simulink model "FourFlexibleBarsFreeAug"  (R2025b)
settings: Solver=VariableStepAuto  StartTime=0.0  StopTime=10.0  RelTol=1e-3
undefined symbols (not defined in the file): E, Iy, Iz, Jr, l0, l1, l2, l3, ni, rho, S, sig4, Theta, uss, xi
libraries: RCTblocks x132
(part 1 of 2)
settings Model: Creator=d.alazard  LastModifiedBy=andre
settings SolverCC: AlgebraicLoopSolver=TrustRegion
settings OptimizationCC: DefaultParameterBehavior=Inlined  BufferReuse=off
settings DebuggingCC: AlgebraicLoopMsg=none  UnconnectedInputMsg=warning  UnconnectedOutputMsg=warning  UnconnectedLineMsg=warning  InitInArrayFormatMsg=none
settings ModelReferenceCC: EnableRefExpFcnMdlSchedulingChecks=on
settings RTWCC: GPUComputeCapability=3.5  DLArmComputeVersion=19.05

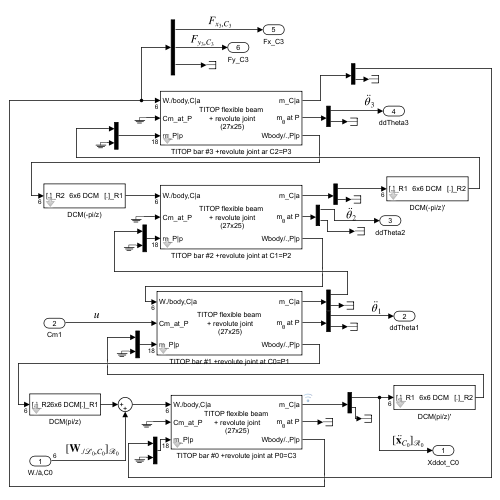
[thumbnail: Simulink's stored preview of the top-level diagram]
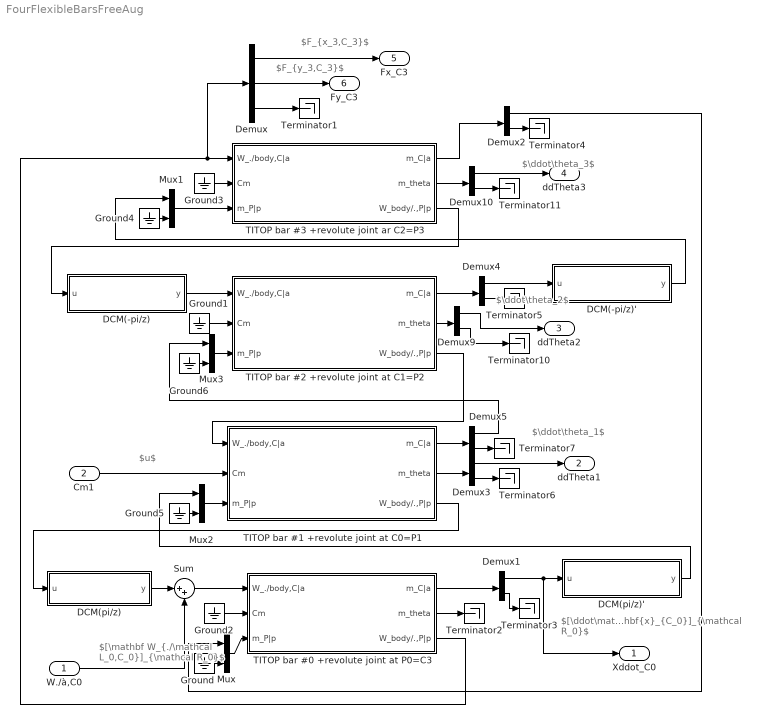
== system FourFlexibleBarsFreeAug ==
  note: $[\mathbf W_{./\mathcal L_0,C_0}]_{\mathcal R_0}$
  note: $\ddot\theta_1$
  note: $u$
  note: $\ddot\theta_2$
  note: $\ddot\theta_3$
  note: $F_{x_3,C_3}$
  note: $F_{y_3,C_3}$
  note: $[\ddot\mathbf{x}_{C_0}]_{\mathcal R_0}$
  W./à,C0 : Inport  PortDimensions=6
  Cm1 : Inport  Port=2
  DCM(-pi/z) : Subsystem  mask(6x6 Direction cosine matrix (DCM)){rot=[-1 0 0;0 -1 0;0 0 1], transp=off}
      mask prompts: rot "3x3 DCM"; transp "Matrix transposed"
      mask help:
      | For 6 d.o.f. body motion (3 translations and 3 rotations), this block Implement the 6x6 rotation matrix (or its transposed) for a given 3x3 DCM.
      |
      | Considering 2 frames R1 and  R2, the DCM between R1 and R2 is defined as the 3x3 matrix where each column is the component vector of each R2 orthogonal unit vector expressed in R1. Thus
      |
      |    [v]_R1 = DCM  * [v]_R2.
      mask init:
      | if transp,
      |     rot=rot';
      | end
      mask Help: web('Doc6dcm.html','-browser')
      mask Display:
      | disp('6x6 DCM')
      | if transp
      |     port_label('input', 1, '[.]_R1')
      |     port_label('output', 1, '[.]_R2')
      | else
      |     port_label('input', 1, '[.]_R2')
      |     port_label('output', 1, '[.]_R1')
      | end
  DCM(-pi/z)' : Subsystem  mask(6x6 Direction cosine matrix (DCM)){rot=[-1 0 0;0 -1 0;0 0 1], transp=on}
      mask prompts: rot "3x3 DCM"; transp "Matrix transposed"
      mask help:
      | For 6 d.o.f. body motion (3 translations and 3 rotations), this block Implement the 6x6 rotation matrix (or its transposed) for a given 3x3 DCM.
      |
      | Considering 2 frames R1 and  R2, the DCM between R1 and R2 is defined as the 3x3 matrix where each column is the component vector of each R2 orthogonal unit vector expressed in R1. Thus
      |
      |    [v]_R1 = DCM  * [v]_R2.
      mask init:
      | if transp,
      |     rot=rot';
      | end
      mask Help: web('Doc6dcm.html','-browser')
      mask Display:
      | disp('6x6 DCM')
      | if transp
      |     port_label('input', 1, '[.]_R1')
      |     port_label('output', 1, '[.]_R2')
      | else
      |     port_label('input', 1, '[.]_R2')
      |     port_label('output', 1, '[.]_R1')
      | end
  DCM(pi/z) : Subsystem  mask(6x6 Direction cosine matrix (DCM)){rot=[-1 0 0;0 -1 0;0 0 1], transp=off}
      mask prompts: rot "3x3 DCM"; transp "Matrix transposed"
      mask help:
      | For 6 d.o.f. body motion (3 translations and 3 rotations), this block Implement the 6x6 rotation matrix (or its transposed) for a given 3x3 DCM.
      |
      | Considering 2 frames R1 and  R2, the DCM between R1 and R2 is defined as the 3x3 matrix where each column is the component vector of each R2 orthogonal unit vector expressed in R1. Thus
      |
      |    [v]_R1 = DCM  * [v]_R2.
      mask init:
      | if transp,
      |     rot=rot';
      | end
      mask Help: web('Doc6dcm.html','-browser')
      mask Display:
      | disp('6x6 DCM')
      | if transp
      |     port_label('input', 1, '[.]_R1')
      |     port_label('output', 1, '[.]_R2')
      | else
      |     port_label('input', 1, '[.]_R2')
      |     port_label('output', 1, '[.]_R1')
      | end
  DCM(pi/z)' : Subsystem  mask(6x6 Direction cosine matrix (DCM)){rot=[-1 0 0;0 -1 0;0 0 1], transp=on}
      mask prompts: rot "3x3 DCM"; transp "Matrix transposed"
      mask help:
      | For 6 d.o.f. body motion (3 translations and 3 rotations), this block Implement the 6x6 rotation matrix (or its transposed) for a given 3x3 DCM.
      |
      | Considering 2 frames R1 and  R2, the DCM between R1 and R2 is defined as the 3x3 matrix where each column is the component vector of each R2 orthogonal unit vector expressed in R1. Thus
      |
      |    [v]_R1 = DCM  * [v]_R2.
      mask init:
      | if transp,
      |     rot=rot';
      | end
      mask Help: web('Doc6dcm.html','-browser')
      mask Display:
      | disp('6x6 DCM')
      | if transp
      |     port_label('input', 1, '[.]_R1')
      |     port_label('output', 1, '[.]_R2')
      | else
      |     port_label('input', 1, '[.]_R2')
      |     port_label('output', 1, '[.]_R1')
      | end
  Demux : Demux  Outputs=[1 1 4]
  Demux{1..2,4..5} (4 alike) : Demux  Outputs=[6 12]
  Demux10 : Demux  Outputs=[1 2]
  Demux3 : Demux  Outputs=[1 2]
  Demux9 : Demux  Outputs=[1 2]
  Ground{,1..6} (7 alike) : Ground
  Mux{,1..3} (4 alike) : Mux  Inputs=[6 12]
  Sum : Sum  Inputs=|++
  TITOP bar #0 +revolute joint at P0=C3 : Subsystem  mask(TITOP flexible beam with revolute joint (27x25)){l=l0, s=S, rho=rho, E=E, Iz=Iz, Iy=Iy, ni=ni, xi=xi, Won=off, uw_var=0, Nflex=0, ra=[0;0;-1], theta=Theta}
      mask prompts: l "length along x (m)"; s "cross section (m^2)"; rho "mass density (Kg/m^3)"; E "Young modulus (N/m^2)"; Iz "second moment of area along z axis, Iz (m^4)"; Iy "second moment of area along y axis Iy, (m^4)"; ni "Poisson coefficient"; xi "dampig ratio"; uw_var "uncertainty (d_w, %)"; Nflex "number of flexible mode (Nflex, integer<=10)"; ra "ra (joint axis) (3x1 vector)"; theta "angular configuration (rad)"
      mask help:
      | Computes the 27x25 model :
      | - 18x6 transfer from the wrenches applied to this body to the motion vector at port C,
      | - the 3x1 channel:
      |               * from  the  joint torque applied by the input (parent) shaft to the output (body) shaft
      |               * to the relative motion vector of the output shaft w.r.t the input shaft [thetaddot;thetadot;theta].
      | - 6x18 transfer from the motion vector to the wrench applied by this body to a parent body at port P through a revolute joint
      |
      | Input/Output of port P are expressed in the parent frame Rp
      | Input/Output of port C are expressed in the body frame Ra.
      |
      | ra: direction of the revolute joint in the Rp (or Ra)
      | theta: angular configuration of the joint (Ra is obtained from Rp by a rotation of theta around ra).
      |
      | All parameters must be expressed in the body frame Ra.
      | Each parameter can be an uncertain parameter declared with the function ureal (except ra)
      |
      | Rk: if "theta" field is: ureal('NAME',0,'Range',[-pi pi])
      | then, ULINEARIZE will provide a model involving the block named "tan_NAME_div4";
      mask init:
      | BeamRev2PortAug
      mask Help: web('DocBeamRevolute.html','-browser')
      mask DialogControl Container5 Prompt: Direct uncertainties on flexible mode frequencies
      mask DialogControl Control2 Prompt: Uncertainties on physical parameters (length, mass, ..) can create huge LFTs.
      mask DialogControl Control3 Prompt: Check this box to overwrite physical parameter uncertainties by a common relative uncertainty (d_w, %) on the first (Nflex) flexible mode frequencies of the clamped at P / free at C beam.
      mask DialogControl Control4 Prompt: The uncertain frequency is named: 'w_name_i' where:
      mask DialogControl Control5 Prompt: * 'name' is the current block name (reduced to its alphanumeric characters).
      mask DialogControl Control6 Prompt: * 'i' is the flexible mode number (increasing frequency order)
      mask DialogControl Container6 Prompt: Joint data
      mask Display:
      | disp('TITOP flexible beam\n + revolute joint\n (27x25)')
      | 
      | port_label('input', 1,'W./body,C|a')
      | port_label('output',1,'m_C|a')
      | port_label('input', 2,'Cm_at_P')
      | port_label('output',2,'m_\theta at P','interpreter','tex')
      | port_label('input', 3,'m_P|p')
      | port_label('output',3,'Wbody/.,P|p')
  TITOP bar #1 +revolute joint at C0=P1 : Subsystem  mask(TITOP flexible beam with revolute joint (27x25)){l=l1, s=S, rho=rho, E=E, Iz=Iz, Iy=Iy, ni=ni, xi=xi, Won=off, uw_var=0, Nflex=0, ra=[0;0;1], theta=Theta}
      mask prompts: l "length along x (m)"; s "cross section (m^2)"; rho "mass density (Kg/m^3)"; E "Young modulus (N/m^2)"; Iz "second moment of area along z axis, Iz (m^4)"; Iy "second moment of area along y axis Iy, (m^4)"; ni "Poisson coefficient"; xi "dampig ratio"; uw_var "uncertainty (d_w, %)"; Nflex "number of flexible mode (Nflex, integer<=10)"; ra "ra (joint axis) (3x1 vector)"; theta "angular configuration (rad)"
      mask help:
      | Computes the 27x25 model :
      | - 18x6 transfer from the wrenches applied to this body to the motion vector at port C,
      | - the 3x1 channel:
      |               * from  the  joint torque applied by the input (parent) shaft to the output (body) shaft
      |               * to the relative motion vector of the output shaft w.r.t the input shaft [thetaddot;thetadot;theta].
      | - 6x18 transfer from the motion vector to the wrench applied by this body to a parent body at port P through a revolute joint
      |
      | Input/Output of port P are expressed in the parent frame Rp
      | Input/Output of port C are expressed in the body frame Ra.
      |
      | ra: direction of the revolute joint in the Rp (or Ra)
      | theta: angular configuration of the joint (Ra is obtained from Rp by a rotation of theta around ra).
      |
      | All parameters must be expressed in the body frame Ra.
      | Each parameter can be an uncertain parameter declared with the function ureal (except ra)
      |
      | Rk: if "theta" field is: ureal('NAME',0,'Range',[-pi pi])
      | then, ULINEARIZE will provide a model involving the block named "tan_NAME_div4";
      mask init:
      | BeamRev2PortAug
      mask Help: web('DocBeamRevolute.html','-browser')
      mask DialogControl Container5 Prompt: Direct uncertainties on flexible mode frequencies
      mask DialogControl Control2 Prompt: Uncertainties on physical parameters (length, mass, ..) can create huge LFTs.
      mask DialogControl Control3 Prompt: Check this box to overwrite physical parameter uncertainties by a common relative uncertainty (d_w, %) on the first (Nflex) flexible mode frequencies of the clamped at P / free at C beam.
      mask DialogControl Control4 Prompt: The uncertain frequency is named: 'w_name_i' where:
      mask DialogControl Control5 Prompt: * 'name' is the current block name (reduced to its alphanumeric characters).
      mask DialogControl Control6 Prompt: * 'i' is the flexible mode number (increasing frequency order)
      mask DialogControl Container6 Prompt: Joint data
      mask Display:
      | disp('TITOP flexible beam\n + revolute joint\n (27x25)')
      | 
      | port_label('input', 1,'W./body,C|a')
      | port_label('output',1,'m_C|a')
      | port_label('input', 2,'Cm_at_P')
      | port_label('output',2,'m_\theta at P','interpreter','tex')
      | port_label('input', 3,'m_P|p')
      | port_label('output',3,'Wbody/.,P|p')
  TITOP bar #2 +revolute joint at C1=P2 : Subsystem  mask(TITOP flexible beam with revolute joint (27x25)){l=l2, s=S, rho=rho, E=E, Iz=Iz, Iy=Iy, ni=ni, xi=xi, Won=off, uw_var=0, Nflex=0, ra=[0;0;-1], theta=Theta}
      mask prompts: l "length along x (m)"; s "cross section (m^2)"; rho "mass density (Kg/m^3)"; E "Young modulus (N/m^2)"; Iz "second moment of area along z axis, Iz (m^4)"; Iy "second moment of area along y axis Iy, (m^4)"; ni "Poisson coefficient"; xi "dampig ratio"; uw_var "uncertainty (d_w, %)"; Nflex "number of flexible mode (Nflex, integer<=10)"; ra "ra (joint axis) (3x1 vector)"; theta "angular configuration (rad)"
      mask help:
      | Computes the 27x25 model :
      | - 18x6 transfer from the wrenches applied to this body to the motion vector at port C,
      | - the 3x1 channel:
      |               * from  the  joint torque applied by the input (parent) shaft to the output (body) shaft
      |               * to the relative motion vector of the output shaft w.r.t the input shaft [thetaddot;thetadot;theta].
      | - 6x18 transfer from the motion vector to the wrench applied by this body to a parent body at port P through a revolute joint
      |
      | Input/Output of port P are expressed in the parent frame Rp
      | Input/Output of port C are expressed in the body frame Ra.
      |
      | ra: direction of the revolute joint in the Rp (or Ra)
      | theta: angular configuration of the joint (Ra is obtained from Rp by a rotation of theta around ra).
      |
      | All parameters must be expressed in the body frame Ra.
      | Each parameter can be an uncertain parameter declared with the function ureal (except ra)
      |
      | Rk: if "theta" field is: ureal('NAME',0,'Range',[-pi pi])
      | then, ULINEARIZE will provide a model involving the block named "tan_NAME_div4";
      mask init:
      | BeamRev2PortAug
      mask Help: web('DocBeamRevolute.html','-browser')
      mask DialogControl Container5 Prompt: Direct uncertainties on flexible mode frequencies
      mask DialogControl Control2 Prompt: Uncertainties on physical parameters (length, mass, ..) can create huge LFTs.
      mask DialogControl Control3 Prompt: Check this box to overwrite physical parameter uncertainties by a common relative uncertainty (d_w, %) on the first (Nflex) flexible mode frequencies of the clamped at P / free at C beam.
      mask DialogControl Control4 Prompt: The uncertain frequency is named: 'w_name_i' where:
      mask DialogControl Control5 Prompt: * 'name' is the current block name (reduced to its alphanumeric characters).
      mask DialogControl Control6 Prompt: * 'i' is the flexible mode number (increasing frequency order)
      mask DialogControl Container6 Prompt: Joint data
      mask Display:
      | disp('TITOP flexible beam\n + revolute joint\n (27x25)')
      | 
      | port_label('input', 1,'W./body,C|a')
      | port_label('output',1,'m_C|a')
      | port_label('input', 2,'Cm_at_P')
      | port_label('output',2,'m_\theta at P','interpreter','tex')
      | port_label('input', 3,'m_P|p')
      | port_label('output',3,'Wbody/.,P|p')
  TITOP bar #3 +revolute joint ar C2=P3 : Subsystem  mask(TITOP flexible beam with revolute joint (27x25)){l=l3, s=S, rho=rho, E=E, Iz=Iz, Iy=Iy, ni=ni, xi=xi, Won=off, uw_var=0, Nflex=0, ra=[0;0;1], theta=Theta}
      mask prompts: l "length along x (m)"; s "cross section (m^2)"; rho "mass density (Kg/m^3)"; E "Young modulus (N/m^2)"; Iz "second moment of area along z axis, Iz (m^4)"; Iy "second moment of area along y axis Iy, (m^4)"; ni "Poisson coefficient"; xi "dampig ratio"; uw_var "uncertainty (d_w, %)"; Nflex "number of flexible mode (Nflex, integer<=10)"; ra "ra (joint axis) (3x1 vector)"; theta "angular configuration (rad)"
      mask help:
      | Computes the 27x25 model :
      | - 18x6 transfer from the wrenches applied to this body to the motion vector at port C,
      | - the 3x1 channel:
      |               * from  the  joint torque applied by the input (parent) shaft to the output (body) shaft
      |               * to the relative motion vector of the output shaft w.r.t the input shaft [thetaddot;thetadot;theta].
      | - 6x18 transfer from the motion vector to the wrench applied by this body to a parent body at port P through a revolute joint
      |
      | Input/Output of port P are expressed in the parent frame Rp
      | Input/Output of port C are expressed in the body frame Ra.
      |
      | ra: direction of the revolute joint in the Rp (or Ra)
      | theta: angular configuration of the joint (Ra is obtained from Rp by a rotation of theta around ra).
      |
      | All parameters must be expressed in the body frame Ra.
      | Each parameter can be an uncertain parameter declared with the function ureal (except ra)
      |
      | Rk: if "theta" field is: ureal('NAME',0,'Range',[-pi pi])
      | then, ULINEARIZE will provide a model involving the block named "tan_NAME_div4";
      mask init:
      | BeamRev2PortAug
      mask Help: web('DocBeamRevolute.html','-browser')
      mask DialogControl Container5 Prompt: Direct uncertainties on flexible mode frequencies
      mask DialogControl Control2 Prompt: Uncertainties on physical parameters (length, mass, ..) can create huge LFTs.
      mask DialogControl Control3 Prompt: Check this box to overwrite physical parameter uncertainties by a common relative uncertainty (d_w, %) on the first (Nflex) flexible mode frequencies of the clamped at P / free at C beam.
      mask DialogControl Control4 Prompt: The uncertain frequency is named: 'w_name_i' where:
      mask DialogControl Control5 Prompt: * 'name' is the current block name (reduced to its alphanumeric characters).
      mask DialogControl Control6 Prompt: * 'i' is the flexible mode number (increasing frequency order)
      mask DialogControl Container6 Prompt: Joint data
      mask Display:
      | disp('TITOP flexible beam\n + revolute joint\n (27x25)')
      | 
      | port_label('input', 1,'W./body,C|a')
      | port_label('output',1,'m_C|a')
      | port_label('input', 2,'Cm_at_P')
      | port_label('output',2,'m_\theta at P','interpreter','tex')
      | port_label('input', 3,'m_P|p')
      | port_label('output',3,'Wbody/.,P|p')
  Terminator{1..7,10..11} (9 alike) : Terminator
  Xddot_C0 : Outport
  ddTheta1 : Outport  Port=2
  ddTheta2 : Outport  Port=3
  ddTheta3 : Outport  Port=4
  Fx_C3 : Outport  Port=5
  Fy_C3 : Outport  Port=6
  wires:
  Ground1/1 -> TITOP bar #2 +revolute joint at C1=P2/2(Cm)
  Demux3/1 -> ddTheta1/1
  Demux9/1 -> ddTheta2/1
  Cm1/1 -> TITOP bar #1 +revolute joint at C0=P1/2(Cm)
  TITOP bar #3 +revolute joint ar C2=P3/3(W_body/.,P|p) -> DCM(-pi/z)/1(u)
  TITOP bar #0 +revolute joint at P0=C3/1(m_C|a) -> Demux1/1
  DCM(-pi/z)/1(y) -> TITOP bar #2 +revolute joint at C1=P2/1(W_./body,C|a)
  TITOP bar #2 +revolute joint at C1=P2/3(W_body/.,P|p) -> TITOP bar #1 +revolute joint at C0=P1/1(W_./body,C|a)
  Ground2/1 -> TITOP bar #0 +revolute joint at P0=C3/2(Cm)
  TITOP bar #0 +revolute joint at P0=C3/2(m_theta) -> Terminator2/1
  Ground3/1 -> TITOP bar #3 +revolute joint ar C2=P3/2(Cm)
  TITOP bar #0 +revolute joint at P0=C3/3(W_body/.,P|p) -> TITOP bar #3 +revolute joint ar C2=P3/1(W_./body,C|a), Demux/1
  Demux10/1 -> ddTheta3/1
  W./à,C0/1 -> Sum/2
  Sum/1 -> TITOP bar #0 +revolute joint at P0=C3/1(W_./body,C|a)
  Demux/1 -> Fx_C3/1
  Demux/2 -> Fy_C3/1
  Demux/3 -> Terminator1/1
  DCM(pi/z)/1(y) -> Sum/1
  TITOP bar #1 +revolute joint at C0=P1/3(W_body/.,P|p) -> DCM(pi/z)/1(u)
  Demux3/2 -> Terminator6/1
  TITOP bar #1 +revolute joint at C0=P1/2(m_theta) -> Demux3/1
  Demux9/2 -> Terminator10/1
  TITOP bar #2 +revolute joint at C1=P2/2(m_theta) -> Demux9/1
  Demux10/2 -> Terminator11/1
  TITOP bar #3 +revolute joint ar C2=P3/2(m_theta) -> Demux10/1
  Demux1/2 -> Terminator3/1
  Demux2/2 -> Terminator4/1
  TITOP bar #3 +revolute joint ar C2=P3/1(m_C|a) -> Demux2/1
  Demux4/2 -> Terminator5/1
  TITOP bar #2 +revolute joint at C1=P2/1(m_C|a) -> Demux4/1
  Demux4/1 -> DCM(-pi/z)'/1(u)
  Ground/1 -> Mux/2
  Ground4/1 -> Mux1/2
  Mux1/1 -> TITOP bar #3 +revolute joint ar C2=P3/3(m_P|p)
  DCM(-pi/z)'/1(y) -> Mux1/1
  Mux/1 -> TITOP bar #0 +revolute joint at P0=C3/3(m_P|p)
  Demux2/1 -> Mux/1
  Demux1/1 -> Xddot_C0/1, DCM(pi/z)'/1(u)
  Ground5/1 -> Mux2/2
  Mux2/1 -> TITOP bar #1 +revolute joint at C0=P1/3(m_P|p)
  DCM(pi/z)'/1(y) -> Mux2/1
  Ground6/1 -> Mux3/2
  Mux3/1 -> TITOP bar #2 +revolute joint at C1=P2/3(m_P|p)
  Demux5/2 -> Terminator7/1
  TITOP bar #1 +revolute joint at C0=P1/1(m_C|a) -> Demux5/1
  Demux5/1 -> Mux3/1

== system FourFlexibleBarsFreeAug/DCM(-pi//z) ==
  u : Inport  PortDimensions=6
  Demux : Demux  Outputs=[3 3]
  Mux : Mux  Inputs=[3 3]
  rotation : Gain  Gain=rot  Multiplication=Matrix(K*u) (u vector)
  translation : Gain  Gain=rot  Multiplication=Matrix(K*u) (u vector)
  y : Outport  VectorParamsAs1DForOutWhenUnconnected=off
  wires:
  rotation/1 -> Mux/2
  translation/1 -> Mux/1
  Demux/1 -> translation/1
  u/1 -> Demux/1
  Mux/1 -> y/1
  Demux/2 -> rotation/1

== system FourFlexibleBarsFreeAug/DCM(-pi//z)' ==
  u : Inport  PortDimensions=6
  Demux : Demux  Outputs=[3 3]
  Mux : Mux  Inputs=[3 3]
  rotation : Gain  Gain=rot  Multiplication=Matrix(K*u) (u vector)
  translation : Gain  Gain=rot  Multiplication=Matrix(K*u) (u vector)
  y : Outport  VectorParamsAs1DForOutWhenUnconnected=off
  wires:
  Demux/2 -> rotation/1
  Mux/1 -> y/1
  u/1 -> Demux/1
  Demux/1 -> translation/1
  translation/1 -> Mux/1
  rotation/1 -> Mux/2

== system FourFlexibleBarsFreeAug/DCM(pi//z) ==
  u : Inport  PortDimensions=6
  Demux : Demux  Outputs=[3 3]
  Mux : Mux  Inputs=[3 3]
  rotation : Gain  Gain=rot  Multiplication=Matrix(K*u) (u vector)
  translation : Gain  Gain=rot  Multiplication=Matrix(K*u) (u vector)
  y : Outport  VectorParamsAs1DForOutWhenUnconnected=off
  wires:
  rotation/1 -> Mux/2
  translation/1 -> Mux/1
  Demux/1 -> translation/1
  u/1 -> Demux/1
  Mux/1 -> y/1
  Demux/2 -> rotation/1

== system FourFlexibleBarsFreeAug/DCM(pi//z)' ==
  u : Inport  PortDimensions=6
  Demux : Demux  Outputs=[3 3]
  Mux : Mux  Inputs=[3 3]
  rotation : Gain  Gain=rot  Multiplication=Matrix(K*u) (u vector)
  translation : Gain  Gain=rot  Multiplication=Matrix(K*u) (u vector)
  y : Outport  VectorParamsAs1DForOutWhenUnconnected=off
  wires:
  rotation/1 -> Mux/2
  translation/1 -> Mux/1
  Demux/1 -> translation/1
  u/1 -> Demux/1
  Mux/1 -> y/1
  Demux/2 -> rotation/1

== system FourFlexibleBarsFreeAug/TITOP bar #0 +revolute joint at P0=C3 ==
  W_./body,C|a : Inport  PortDimensions=6
  Cm : Inport  Port=2
  m_P|p : Inport  Port=3  PortDimensions=18
  Demux : Demux  Outputs=[18 6]
      settings: DisplayOption=none
  Mux : Mux  Inputs=[6 18]
  Revolute joint + configuration : Subsystem  mask(Revolute joint){ra=ra, Jr=Jr, theta=theta}
      mask prompts: ra "Direction of the joint in the local frame (3x1 vector)"; Jr "Rotor inertia (kg.m^2)"; theta "Angular configuration (rad)"
      mask help:
      | This block implement the TITOP model of of a revolute joint.
      | The last channel is the transfer between the torque applied inside the joint by the input shaft to the output shaft and the relative angular acceleration of the output shaft w.r.t the input shaft.
      |
      | Angular configuration can be a vayring parameter: Ex:
      | ureal('NAME',0,'Range',[-pi pi])
      |
      | Then, ULINEARIZE will provide a model involving the block named "tan_NAME_div4";
      mask init:
      | pass=ra2DCMi(ra);
      | ran=[ra(1);ra(2);ra(3)]/norm(ra);
      mask Help: web('DocRevoluteJoint_configuration.html','-browser')
      mask Display:
      | disp('Revolute joint\nTITOP model\n+ angle configuration')
      | port_label('input', 1, 'W_./r_out|a')
      | port_label('output', 1, 'm_out|a')
      | port_label('input', 2, 'm_in|p')
      | port_label('output', 2, 'W_r_in/.|p')
      | port_label('input', 3, 'Cm')
      | port_label('output', 3, 'm_\theta','interpreter','tex')
  Uncertain State Space : RCTblocks/Uncertain State Space  Tag=USS  USystem=TITOPBEAM  UValue=[]  X0=[]  uX0=[]
  m_C|a : Outport  VectorParamsAs1DForOutWhenUnconnected=off
  m_theta : Outport  Port=2  VectorParamsAs1DForOutWhenUnconnected=off
  W_body/.,P|p : Outport  Port=3  VectorParamsAs1DForOutWhenUnconnected=off
  wires:
  Cm/1 -> Revolute joint + configuration/3(Cm)
  Revolute joint + configuration/1(m_out|a) -> Mux/2
  Revolute joint + configuration/2(W_r_in/.|p) -> W_body/.,P|p/1
  Revolute joint + configuration/3(m_theta) -> m_theta/1
  m_P|p/1 -> Revolute joint + configuration/2(m_in|p)
  Demux/2 -> Revolute joint + configuration/1(W_./r_out|a)
  Demux/1 -> m_C|a/1
  W_./body,C|a/1 -> Mux/1
  Mux/1 -> Uncertain State Space/1
  Uncertain State Space/1 -> Demux/1

== system FourFlexibleBarsFreeAug/TITOP bar #1 +revolute joint at C0=P1 ==
  W_./body,C|a : Inport  PortDimensions=6
  Cm : Inport  Port=2
  m_P|p : Inport  Port=3  PortDimensions=18
  Demux : Demux  Outputs=[18 6]
      settings: DisplayOption=none
  Mux : Mux  Inputs=[6 18]
  Revolute joint + configuration : Subsystem  mask(Revolute joint){ra=ra, Jr=Jr, theta=theta}
      mask prompts: ra "Direction of the joint in the local frame (3x1 vector)"; Jr "Rotor inertia (kg.m^2)"; theta "Angular configuration (rad)"
      mask help:
      | This block implement the TITOP model of of a revolute joint.
      | The last channel is the transfer between the torque applied inside the joint by the input shaft to the output shaft and the relative angular acceleration of the output shaft w.r.t the input shaft.
      |
      | Angular configuration can be a vayring parameter: Ex:
      | ureal('NAME',0,'Range',[-pi pi])
      |
      | Then, ULINEARIZE will provide a model involving the block named "tan_NAME_div4";
      mask init:
      | pass=ra2DCMi(ra);
      | ran=[ra(1);ra(2);ra(3)]/norm(ra);
      mask Help: web('DocRevoluteJoint_configuration.html','-browser')
      mask Display:
      | disp('Revolute joint\nTITOP model\n+ angle configuration')
      | port_label('input', 1, 'W_./r_out|a')
      | port_label('output', 1, 'm_out|a')
      | port_label('input', 2, 'm_in|p')
      | port_label('output', 2, 'W_r_in/.|p')
      | port_label('input', 3, 'Cm')
      | port_label('output', 3, 'm_\theta','interpreter','tex')
  Uncertain State Space : RCTblocks/Uncertain State Space  Tag=USS  USystem=TITOPBEAM  UValue=[]  X0=[]  uX0=[]
  m_C|a : Outport  VectorParamsAs1DForOutWhenUnconnected=off
  m_theta : Outport  Port=2  VectorParamsAs1DForOutWhenUnconnected=off
  W_body/.,P|p : Outport  Port=3  VectorParamsAs1DForOutWhenUnconnected=off
  wires:
  Uncertain State Space/1 -> Demux/1
  Mux/1 -> Uncertain State Space/1
  W_./body,C|a/1 -> Mux/1
  Demux/1 -> m_C|a/1
  Demux/2 -> Revolute joint + configuration/1(W_./r_out|a)
  m_P|p/1 -> Revolute joint + configuration/2(m_in|p)
  Revolute joint + configuration/3(m_theta) -> m_theta/1
  Revolute joint + configuration/2(W_r_in/.|p) -> W_body/.,P|p/1
  Revolute joint + configuration/1(m_out|a) -> Mux/2
  Cm/1 -> Revolute joint + configuration/3(Cm)

== system FourFlexibleBarsFreeAug/TITOP bar #2 +revolute joint at C1=P2 ==
  W_./body,C|a : Inport  PortDimensions=6
  Cm : Inport  Port=2
  m_P|p : Inport  Port=3  PortDimensions=18
  Demux : Demux  Outputs=[18 6]
      settings: DisplayOption=none
  Mux : Mux  Inputs=[6 18]
  Revolute joint + configuration : Subsystem  mask(Revolute joint){ra=ra, Jr=Jr, theta=theta}
      mask prompts: ra "Direction of the joint in the local frame (3x1 vector)"; Jr "Rotor inertia (kg.m^2)"; theta "Angular configuration (rad)"
      mask help:
      | This block implement the TITOP model of of a revolute joint.
      | The last channel is the transfer between the torque applied inside the joint by the input shaft to the output shaft and the relative angular acceleration of the output shaft w.r.t the input shaft.
      |
      | Angular configuration can be a vayring parameter: Ex:
      | ureal('NAME',0,'Range',[-pi pi])
      |
      | Then, ULINEARIZE will provide a model involving the block named "tan_NAME_div4";
      mask init:
      | pass=ra2DCMi(ra);
      | ran=[ra(1);ra(2);ra(3)]/norm(ra);
      mask Help: web('DocRevoluteJoint_configuration.html','-browser')
      mask Display:
      | disp('Revolute joint\nTITOP model\n+ angle configuration')
      | port_label('input', 1, 'W_./r_out|a')
      | port_label('output', 1, 'm_out|a')
      | port_label('input', 2, 'm_in|p')
      | port_label('output', 2, 'W_r_in/.|p')
      | port_label('input', 3, 'Cm')
      | port_label('output', 3, 'm_\theta','interpreter','tex')
  Uncertain State Space : RCTblocks/Uncertain State Space  Tag=USS  USystem=TITOPBEAM  UValue=[]  X0=[]  uX0=[]
  m_C|a : Outport  VectorParamsAs1DForOutWhenUnconnected=off
  m_theta : Outport  Port=2  VectorParamsAs1DForOutWhenUnconnected=off
  W_body/.,P|p : Outport  Port=3  VectorParamsAs1DForOutWhenUnconnected=off
  wires:
  Uncertain State Space/1 -> Demux/1
  Mux/1 -> Uncertain State Space/1
  W_./body,C|a/1 -> Mux/1
  Demux/1 -> m_C|a/1
  Demux/2 -> Revolute joint + configuration/1(W_./r_out|a)
  m_P|p/1 -> Revolute joint + configuration/2(m_in|p)
  Revolute joint + configuration/3(m_theta) -> m_theta/1
  Revolute joint + configuration/2(W_r_in/.|p) -> W_body/.,P|p/1
  Revolute joint + configuration/1(m_out|a) -> Mux/2
  Cm/1 -> Revolute joint + configuration/3(Cm)

== system FourFlexibleBarsFreeAug/TITOP bar #3 +revolute joint ar C2=P3 ==
  W_./body,C|a : Inport  PortDimensions=6
  Cm : Inport  Port=2
  m_P|p : Inport  Port=3  PortDimensions=18
  Demux : Demux  Outputs=[18 6]
      settings: DisplayOption=none
  Mux : Mux  Inputs=[6 18]
  Revolute joint + configuration : Subsystem  mask(Revolute joint){ra=ra, Jr=Jr, theta=theta}
      mask prompts: ra "Direction of the joint in the local frame (3x1 vector)"; Jr "Rotor inertia (kg.m^2)"; theta "Angular configuration (rad)"
      mask help:
      | This block implement the TITOP model of of a revolute joint.
      | The last channel is the transfer between the torque applied inside the joint by the input shaft to the output shaft and the relative angular acceleration of the output shaft w.r.t the input shaft.
      |
      | Angular configuration can be a vayring parameter: Ex:
      | ureal('NAME',0,'Range',[-pi pi])
      |
      | Then, ULINEARIZE will provide a model involving the block named "tan_NAME_div4";
      mask init:
      | pass=ra2DCMi(ra);
      | ran=[ra(1);ra(2);ra(3)]/norm(ra);
      mask Help: web('DocRevoluteJoint_configuration.html','-browser')
      mask Display:
      | disp('Revolute joint\nTITOP model\n+ angle configuration')
      | port_label('input', 1, 'W_./r_out|a')
      | port_label('output', 1, 'm_out|a')
      | port_label('input', 2, 'm_in|p')
      | port_label('output', 2, 'W_r_in/.|p')
      | port_label('input', 3, 'Cm')
      | port_label('output', 3, 'm_\theta','interpreter','tex')
  Uncertain State Space : RCTblocks/Uncertain State Space  Tag=USS  USystem=TITOPBEAM  UValue=[]  X0=[]  uX0=[]
  m_C|a : Outport  VectorParamsAs1DForOutWhenUnconnected=off
  m_theta : Outport  Port=2  VectorParamsAs1DForOutWhenUnconnected=off
  W_body/.,P|p : Outport  Port=3  VectorParamsAs1DForOutWhenUnconnected=off
  wires:
  Cm/1 -> Revolute joint + configuration/3(Cm)
  Revolute joint + configuration/1(m_out|a) -> Mux/2
  Revolute joint + configuration/2(W_r_in/.|p) -> W_body/.,P|p/1
  Revolute joint + configuration/3(m_theta) -> m_theta/1
  m_P|p/1 -> Revolute joint + configuration/2(m_in|p)
  Demux/2 -> Revolute joint + configuration/1(W_./r_out|a)
  Demux/1 -> m_C|a/1
  W_./body,C|a/1 -> Mux/1
  Mux/1 -> Uncertain State Space/1
  Uncertain State Space/1 -> Demux/1

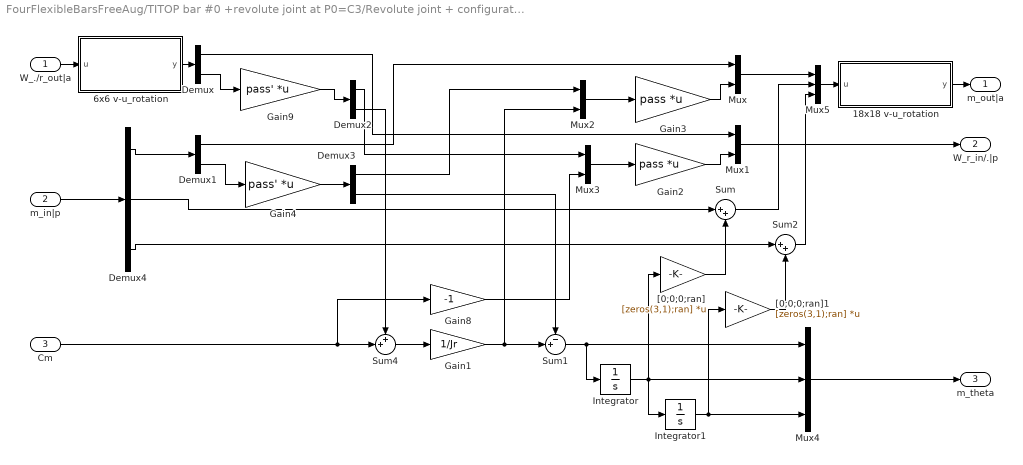
== system FourFlexibleBarsFreeAug/TITOP bar #0 +revolute joint at P0=C3/Revolute joint + configuration ==
  W_./r_out|a : Inport  PortDimensions=6
  m_in|p : Inport  Port=2  PortDimensions=18
  Cm : Inport  Port=3  PortDimensions=1
  18x18 v-u_rotation : Subsystem  mask(18x18 rotation matrix (around a given axis)){ra=ra, theta=theta, transp=on}
      mask prompts: ra "Rotation axis (3x1 vector)"; theta "Angle (rad)"; transp "Matrix transposed"
      mask help:
      | For 6 d.o.f. body motion vector (3 translations and 3 rotations, acceleration velocities and positions), this block Implement the 18x18 rotation matrix (or its transposed)  for a given angle around a given axis.
      |
      | Angle  (rad) can be an uncertain parameter declared with "ureal" with mode 'Range'
      | Ex: ureal('NAME',0,'Range',[-pi pi])
      | Then, ULINEARIZE will provide a model involving the block named "tan_NAME_div4".
      mask init:
      | vUrotation3x3
      mask Help: web('Doc6vurotation.html','-browser')
      mask Display:
      | disp('v-rot\n18x18')
      | if transp
      |     port_label('input', 1, '[.]_R1')
      |     port_label('output', 1, '[.]_R2')
      | else
      |     port_label('input', 1, '[.]_R2')
      |     port_label('output', 1, '[.]_R1')
      | end
  6x6 v-u_rotation : Subsystem  mask(6x6 rotation matrix (around a given axis)){ra=ra, theta=theta, transp=off}
      mask prompts: ra "Rotation axis (3x1 vector)"; theta "Angle (rad)"; transp "Matrix transposed"
      mask help:
      | For 6 d.o.f. body motion (3 translations and 3 rotations), this block Implement the 6x6 rotation matrix (or its transposed) for a given angle around a given axis.
      |
      | Angle  (rad) can be an uncertain parameter declared with "ureal" with mode 'Range'
      | Ex: ureal('NAME',0,'Range',[-pi pi])
      | Then, ULINEARIZE will provide a model involving the block named "tan_NAME_div4".
      mask init:
      | vUrotation3x3
      mask Help: web('Doc6vurotation.html','-browser')
      mask Display:
      | disp('v-rot\n6x6')
      | if transp
      |     port_label('input', 1, '[.]_R1')
      |     port_label('output', 1, '[.]_R2')
      | else
      |     port_label('input', 1, '[.]_R2')
      |     port_label('output', 1, '[.]_R1')
      | end
  Demux : Demux  Outputs=[3 3]
  Demux1 : Demux  Outputs=[3 3]
  Demux2 : Demux  Outputs=[2 1]
  Demux3 : Demux  Outputs=[2 1]
  Demux4 : Demux  Outputs=[6 6 6]
  Gain1 : Gain  Gain=1/Jr
  Gain2 : Gain  Gain=pass  Multiplication=Matrix(K*u) (u vector)
  Gain3 : Gain  Gain=pass  Multiplication=Matrix(K*u) (u vector)
  Gain4 : Gain  Gain=pass'  Multiplication=Matrix(K*u) (u vector)
  Gain8 : Gain  Gain=-1
  Gain9 : Gain  Gain=pass'  Multiplication=Matrix(K*u) (u vector)
  Integrator : Integrator
  Integrator1 : Integrator
  Mux : Mux  Inputs=[3 3]
  Mux1 : Mux  Inputs=[3 3]
  Mux2 : Mux  Inputs=[2 1]
  Mux3 : Mux  Inputs=[2 1]
  Mux4 : Mux  Inputs=3
  Mux5 : Mux  Inputs=[6 6 6]
  Sum : Sum  Inputs=|++
  Sum1 : Sum  Inputs=-+|
  Sum2 : Sum  Inputs=|++
  Sum4 : Sum  Inputs=++|
  "[0;0;0;ran]" : Gain  Gain=[zeros(3,1);ran]  Multiplication=Matrix(K*u) (u vector)
  "[0;0;0;ran]1" : Gain  Gain=[zeros(3,1);ran]  Multiplication=Matrix(K*u) (u vector)
  m_out|a : Outport  VectorParamsAs1DForOutWhenUnconnected=off
  W_r_in/.|p : Outport  Port=2  VectorParamsAs1DForOutWhenUnconnected=off
  m_theta : Outport  Port=3  VectorParamsAs1DForOutWhenUnconnected=off
  wires:
  18x18 v-u_rotation/1(y) -> m_out|a/1
  6x6 v-u_rotation/1(y) -> Demux/1
  Demux3/1 -> Mux2/1
  Demux2/1 -> Mux3/1
  Gain8/1 -> Mux3/2
  Mux3/1 -> Gain2/1
  Gain4/1 -> Demux3/1
  Demux1/2 -> Gain4/1
  Mux2/1 -> Gain3/1
  Demux2/2 -> Sum4/1
  Gain9/1 -> Demux2/1
  Demux3/2 -> Sum1/1
  Gain3/1 -> Mux/2
  Sum4/1 -> Gain1/1
  Gain1/1 -> Sum1/2, Mux2/2
  Demux/2 -> Gain9/1
  Gain2/1 -> Mux1/2
  Demux/1 -> Mux1/1
  Cm/1 -> Sum4/2, Gain8/1
  Demux1/1 -> Mux/1
  Mux1/1 -> W_r_in/.|p/1
  W_./r_out|a/1 -> 6x6 v-u_rotation/1(u)
  Demux4/1 -> Demux1/1
  m_in|p/1 -> Demux4/1
  Integrator/1 -> "[0;0;0;ran]"/1, Mux4/2, Integrator1/1
  Mux4/1 -> m_theta/1
  Sum1/1 -> Integrator/1, Mux4/1
  Integrator1/1 -> "[0;0;0;ran]1"/1, Mux4/3
  "[0;0;0;ran]"/1 -> Sum/2
  "[0;0;0;ran]1"/1 -> Sum2/2
  Demux4/2 -> Sum/1
  Demux4/3 -> Sum2/1
  Mux/1 -> Mux5/1
  Mux5/1 -> 18x18 v-u_rotation/1(u)
  Sum/1 -> Mux5/2
  Sum2/1 -> Mux5/3

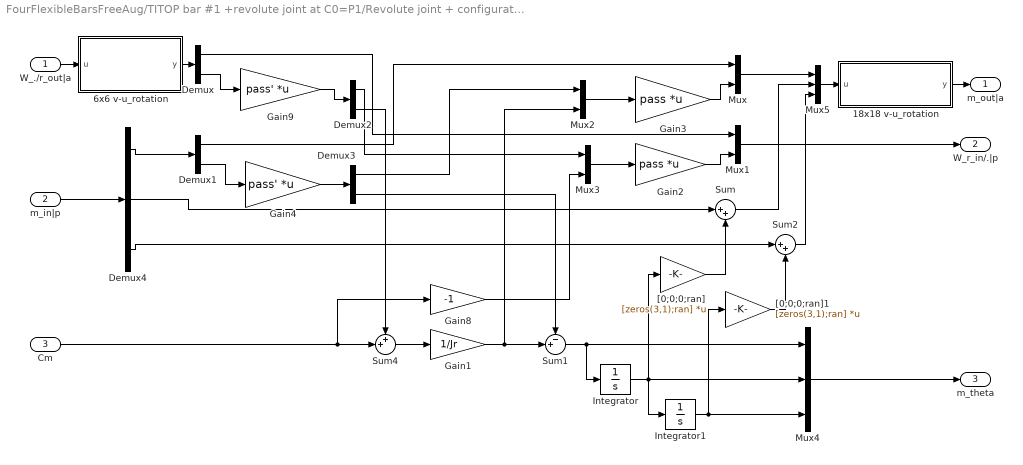
== system FourFlexibleBarsFreeAug/TITOP bar #1 +revolute joint at C0=P1/Revolute joint + configuration ==
  W_./r_out|a : Inport  PortDimensions=6
  m_in|p : Inport  Port=2  PortDimensions=18
  Cm : Inport  Port=3  PortDimensions=1
  18x18 v-u_rotation : Subsystem  mask(18x18 rotation matrix (around a given axis)){ra=ra, theta=theta, transp=on}
      mask prompts: ra "Rotation axis (3x1 vector)"; theta "Angle (rad)"; transp "Matrix transposed"
      mask help:
      | For 6 d.o.f. body motion vector (3 translations and 3 rotations, acceleration velocities and positions), this block Implement the 18x18 rotation matrix (or its transposed)  for a given angle around a given axis.
      |
      | Angle  (rad) can be an uncertain parameter declared with "ureal" with mode 'Range'
      | Ex: ureal('NAME',0,'Range',[-pi pi])
      | Then, ULINEARIZE will provide a model involving the block named "tan_NAME_div4".
      mask init:
      | vUrotation3x3
      mask Help: web('Doc6vurotation.html','-browser')
      mask Display:
      | disp('v-rot\n18x18')
      | if transp
      |     port_label('input', 1, '[.]_R1')
      |     port_label('output', 1, '[.]_R2')
      | else
      |     port_label('input', 1, '[.]_R2')
      |     port_label('output', 1, '[.]_R1')
      | end
  6x6 v-u_rotation : Subsystem  mask(6x6 rotation matrix (around a given axis)){ra=ra, theta=theta, transp=off}
      mask prompts: ra "Rotation axis (3x1 vector)"; theta "Angle (rad)"; transp "Matrix transposed"
      mask help:
      | For 6 d.o.f. body motion (3 translations and 3 rotations), this block Implement the 6x6 rotation matrix (or its transposed) for a given angle around a given axis.
      |
      | Angle  (rad) can be an uncertain parameter declared with "ureal" with mode 'Range'
      | Ex: ureal('NAME',0,'Range',[-pi pi])
      | Then, ULINEARIZE will provide a model involving the block named "tan_NAME_div4".
      mask init:
      | vUrotation3x3
      mask Help: web('Doc6vurotation.html','-browser')
      mask Display:
      | disp('v-rot\n6x6')
      | if transp
      |     port_label('input', 1, '[.]_R1')
      |     port_label('output', 1, '[.]_R2')
      | else
      |     port_label('input', 1, '[.]_R2')
      |     port_label('output', 1, '[.]_R1')
      | end
  Demux : Demux  Outputs=[3 3]
  Demux1 : Demux  Outputs=[3 3]
  Demux2 : Demux  Outputs=[2 1]
  Demux3 : Demux  Outputs=[2 1]
  Demux4 : Demux  Outputs=[6 6 6]
  Gain1 : Gain  Gain=1/Jr
  Gain2 : Gain  Gain=pass  Multiplication=Matrix(K*u) (u vector)
  Gain3 : Gain  Gain=pass  Multiplication=Matrix(K*u) (u vector)
  Gain4 : Gain  Gain=pass'  Multiplication=Matrix(K*u) (u vector)
  Gain8 : Gain  Gain=-1
  Gain9 : Gain  Gain=pass'  Multiplication=Matrix(K*u) (u vector)
  Integrator : Integrator
  Integrator1 : Integrator
  Mux : Mux  Inputs=[3 3]
  Mux1 : Mux  Inputs=[3 3]
  Mux2 : Mux  Inputs=[2 1]
  Mux3 : Mux  Inputs=[2 1]
  Mux4 : Mux  Inputs=3
  Mux5 : Mux  Inputs=[6 6 6]
  Sum : Sum  Inputs=|++
  Sum1 : Sum  Inputs=-+|
  Sum2 : Sum  Inputs=|++
  Sum4 : Sum  Inputs=++|
  "[0;0;0;ran]" : Gain  Gain=[zeros(3,1);ran]  Multiplication=Matrix(K*u) (u vector)
  "[0;0;0;ran]1" : Gain  Gain=[zeros(3,1);ran]  Multiplication=Matrix(K*u) (u vector)
  m_out|a : Outport  VectorParamsAs1DForOutWhenUnconnected=off
  W_r_in/.|p : Outport  Port=2  VectorParamsAs1DForOutWhenUnconnected=off
  m_theta : Outport  Port=3  VectorParamsAs1DForOutWhenUnconnected=off
  wires:
  Sum2/1 -> Mux5/3
  Sum/1 -> Mux5/2
  Mux5/1 -> 18x18 v-u_rotation/1(u)
  Mux/1 -> Mux5/1
  Demux4/3 -> Sum2/1
  Demux4/2 -> Sum/1
  "[0;0;0;ran]1"/1 -> Sum2/2
  "[0;0;0;ran]"/1 -> Sum/2
  Integrator1/1 -> Mux4/3, "[0;0;0;ran]1"/1
  Sum1/1 -> Mux4/1, Integrator/1
  Mux4/1 -> m_theta/1
  Integrator/1 -> Integrator1/1, Mux4/2, "[0;0;0;ran]"/1
  m_in|p/1 -> Demux4/1
  Demux4/1 -> Demux1/1
  W_./r_out|a/1 -> 6x6 v-u_rotation/1(u)
  Mux1/1 -> W_r_in/.|p/1
  Demux1/1 -> Mux/1
  Cm/1 -> Gain8/1, Sum4/2
  Demux/1 -> Mux1/1
  Gain2/1 -> Mux1/2
  Demux/2 -> Gain9/1
  Gain1/1 -> Mux2/2, Sum1/2
  Sum4/1 -> Gain1/1
  Gain3/1 -> Mux/2
  Demux3/2 -> Sum1/1
  Gain9/1 -> Demux2/1
  Demux2/2 -> Sum4/1
  Mux2/1 -> Gain3/1
  Demux1/2 -> Gain4/1
  Gain4/1 -> Demux3/1
  Mux3/1 -> Gain2/1
  Gain8/1 -> Mux3/2
  Demux2/1 -> Mux3/1
  Demux3/1 -> Mux2/1
  6x6 v-u_rotation/1(y) -> Demux/1
  18x18 v-u_rotation/1(y) -> m_out|a/1

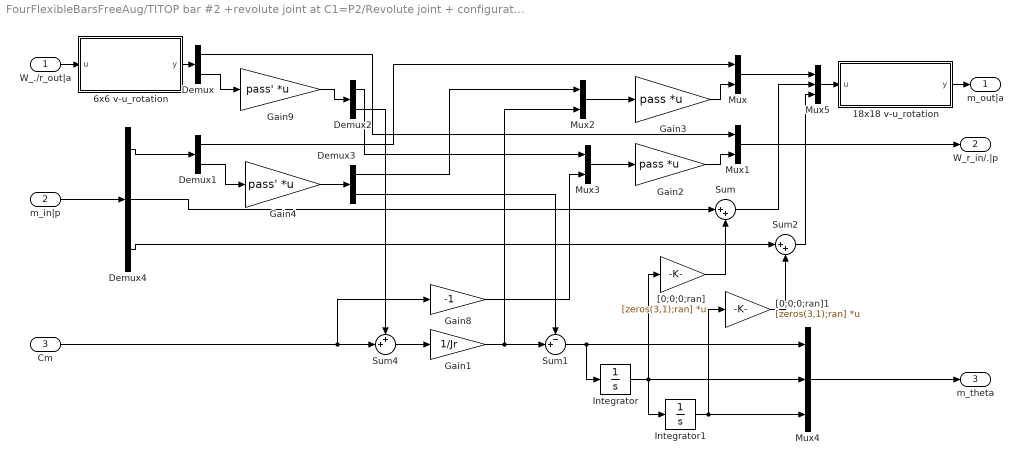
== system FourFlexibleBarsFreeAug/TITOP bar #2 +revolute joint at C1=P2/Revolute joint + configuration ==
  W_./r_out|a : Inport  PortDimensions=6
  m_in|p : Inport  Port=2  PortDimensions=18
  Cm : Inport  Port=3  PortDimensions=1
  18x18 v-u_rotation : Subsystem  mask(18x18 rotation matrix (around a given axis)){ra=ra, theta=theta, transp=on}
      mask prompts: ra "Rotation axis (3x1 vector)"; theta "Angle (rad)"; transp "Matrix transposed"
      mask help:
      | For 6 d.o.f. body motion vector (3 translations and 3 rotations, acceleration velocities and positions), this block Implement the 18x18 rotation matrix (or its transposed)  for a given angle around a given axis.
      |
      | Angle  (rad) can be an uncertain parameter declared with "ureal" with mode 'Range'
      | Ex: ureal('NAME',0,'Range',[-pi pi])
      | Then, ULINEARIZE will provide a model involving the block named "tan_NAME_div4".
      mask init:
      | vUrotation3x3
      mask Help: web('Doc6vurotation.html','-browser')
      mask Display:
      | disp('v-rot\n18x18')
      | if transp
      |     port_label('input', 1, '[.]_R1')
      |     port_label('output', 1, '[.]_R2')
      | else
      |     port_label('input', 1, '[.]_R2')
      |     port_label('output', 1, '[.]_R1')
      | end
  6x6 v-u_rotation : Subsystem  mask(6x6 rotation matrix (around a given axis)){ra=ra, theta=theta, transp=off}
      mask prompts: ra "Rotation axis (3x1 vector)"; theta "Angle (rad)"; transp "Matrix transposed"
      mask help:
      | For 6 d.o.f. body motion (3 translations and 3 rotations), this block Implement the 6x6 rotation matrix (or its transposed) for a given angle around a given axis.
      |
      | Angle  (rad) can be an uncertain parameter declared with "ureal" with mode 'Range'
      | Ex: ureal('NAME',0,'Range',[-pi pi])
      | Then, ULINEARIZE will provide a model involving the block named "tan_NAME_div4".
      mask init:
      | vUrotation3x3
      mask Help: web('Doc6vurotation.html','-browser')
      mask Display:
      | disp('v-rot\n6x6')
      | if transp
      |     port_label('input', 1, '[.]_R1')
      |     port_label('output', 1, '[.]_R2')
      | else
      |     port_label('input', 1, '[.]_R2')
      |     port_label('output', 1, '[.]_R1')
      | end
  Demux : Demux  Outputs=[3 3]
  Demux1 : Demux  Outputs=[3 3]
  Demux2 : Demux  Outputs=[2 1]
  Demux3 : Demux  Outputs=[2 1]
  Demux4 : Demux  Outputs=[6 6 6]
  Gain1 : Gain  Gain=1/Jr
  Gain2 : Gain  Gain=pass  Multiplication=Matrix(K*u) (u vector)
  Gain3 : Gain  Gain=pass  Multiplication=Matrix(K*u) (u vector)
  Gain4 : Gain  Gain=pass'  Multiplication=Matrix(K*u) (u vector)
  Gain8 : Gain  Gain=-1
  Gain9 : Gain  Gain=pass'  Multiplication=Matrix(K*u) (u vector)
  Integrator : Integrator
  Integrator1 : Integrator
  Mux : Mux  Inputs=[3 3]
  Mux1 : Mux  Inputs=[3 3]
  Mux2 : Mux  Inputs=[2 1]
  Mux3 : Mux  Inputs=[2 1]
  Mux4 : Mux  Inputs=3
  Mux5 : Mux  Inputs=[6 6 6]
  Sum : Sum  Inputs=|++
  Sum1 : Sum  Inputs=-+|
  Sum2 : Sum  Inputs=|++
  Sum4 : Sum  Inputs=++|
  "[0;0;0;ran]" : Gain  Gain=[zeros(3,1);ran]  Multiplication=Matrix(K*u) (u vector)
  "[0;0;0;ran]1" : Gain  Gain=[zeros(3,1);ran]  Multiplication=Matrix(K*u) (u vector)
  m_out|a : Outport  VectorParamsAs1DForOutWhenUnconnected=off
  W_r_in/.|p : Outport  Port=2  VectorParamsAs1DForOutWhenUnconnected=off
  m_theta : Outport  Port=3  VectorParamsAs1DForOutWhenUnconnected=off
  wires:
  Sum2/1 -> Mux5/3
  Sum/1 -> Mux5/2
  Mux5/1 -> 18x18 v-u_rotation/1(u)
  Mux/1 -> Mux5/1
  Demux4/3 -> Sum2/1
  Demux4/2 -> Sum/1
  "[0;0;0;ran]1"/1 -> Sum2/2
  "[0;0;0;ran]"/1 -> Sum/2
  Integrator1/1 -> Mux4/3, "[0;0;0;ran]1"/1
  Sum1/1 -> Mux4/1, Integrator/1
  Mux4/1 -> m_theta/1
  Integrator/1 -> Integrator1/1, Mux4/2, "[0;0;0;ran]"/1
  m_in|p/1 -> Demux4/1
  Demux4/1 -> Demux1/1
  W_./r_out|a/1 -> 6x6 v-u_rotation/1(u)
  Mux1/1 -> W_r_in/.|p/1
  Demux1/1 -> Mux/1
  Cm/1 -> Gain8/1, Sum4/2
  Demux/1 -> Mux1/1
  Gain2/1 -> Mux1/2
  Demux/2 -> Gain9/1
  Gain1/1 -> Mux2/2, Sum1/2
  Sum4/1 -> Gain1/1
  Gain3/1 -> Mux/2
  Demux3/2 -> Sum1/1
  Gain9/1 -> Demux2/1
  Demux2/2 -> Sum4/1
  Mux2/1 -> Gain3/1
  Demux1/2 -> Gain4/1
  Gain4/1 -> Demux3/1
  Mux3/1 -> Gain2/1
  Gain8/1 -> Mux3/2
  Demux2/1 -> Mux3/1
  Demux3/1 -> Mux2/1
  6x6 v-u_rotation/1(y) -> Demux/1
  18x18 v-u_rotation/1(y) -> m_out|a/1

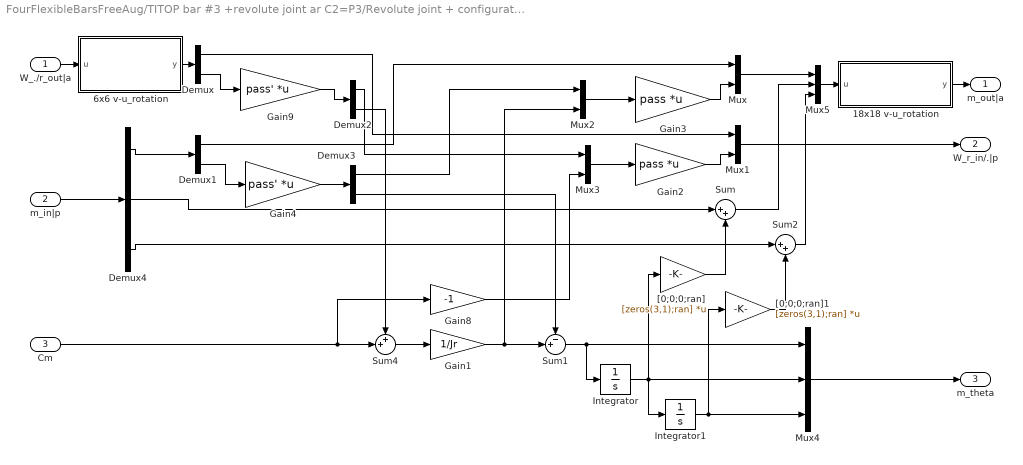
== system FourFlexibleBarsFreeAug/TITOP bar #3 +revolute joint ar C2=P3/Revolute joint + configuration ==
  W_./r_out|a : Inport  PortDimensions=6
  m_in|p : Inport  Port=2  PortDimensions=18
  Cm : Inport  Port=3  PortDimensions=1
  18x18 v-u_rotation : Subsystem  mask(18x18 rotation matrix (around a given axis)){ra=ra, theta=theta, transp=on}
      mask prompts: ra "Rotation axis (3x1 vector)"; theta "Angle (rad)"; transp "Matrix transposed"
      mask help:
      | For 6 d.o.f. body motion vector (3 translations and 3 rotations, acceleration velocities and positions), this block Implement the 18x18 rotation matrix (or its transposed)  for a given angle around a given axis.
      |
      | Angle  (rad) can be an uncertain parameter declared with "ureal" with mode 'Range'
      | Ex: ureal('NAME',0,'Range',[-pi pi])
      | Then, ULINEARIZE will provide a model involving the block named "tan_NAME_div4".
      mask init:
      | vUrotation3x3
      mask Help: web('Doc6vurotation.html','-browser')
      mask Display:
      | disp('v-rot\n18x18')
      | if transp
      |     port_label('input', 1, '[.]_R1')
      |     port_label('output', 1, '[.]_R2')
      | else
      |     port_label('input', 1, '[.]_R2')
      |     port_label('output', 1, '[.]_R1')
      | end
  6x6 v-u_rotation : Subsystem  mask(6x6 rotation matrix (around a given axis)){ra=ra, theta=theta, transp=off}
      mask prompts: ra "Rotation axis (3x1 vector)"; theta "Angle (rad)"; transp "Matrix transposed"
      mask help:
      | For 6 d.o.f. body motion (3 translations and 3 rotations), this block Implement the 6x6 rotation matrix (or its transposed) for a given angle around a given axis.
      |
      | Angle  (rad) can be an uncertain parameter declared with "ureal" with mode 'Range'
      | Ex: ureal('NAME',0,'Range',[-pi pi])
      | Then, ULINEARIZE will provide a model involving the block named "tan_NAME_div4".
      mask init:
      | vUrotation3x3
      mask Help: web('Doc6vurotation.html','-browser')
      mask Display:
      | disp('v-rot\n6x6')
      | if transp
      |     port_label('input', 1, '[.]_R1')
      |     port_label('output', 1, '[.]_R2')
      | else
      |     port_label('input', 1, '[.]_R2')
      |     port_label('output', 1, '[.]_R1')
      | end
  Demux : Demux  Outputs=[3 3]
  Demux1 : Demux  Outputs=[3 3]
  Demux2 : Demux  Outputs=[2 1]
  Demux3 : Demux  Outputs=[2 1]
  Demux4 : Demux  Outputs=[6 6 6]
  Gain1 : Gain  Gain=1/Jr
  Gain2 : Gain  Gain=pass  Multiplication=Matrix(K*u) (u vector)
  Gain3 : Gain  Gain=pass  Multiplication=Matrix(K*u) (u vector)
  Gain4 : Gain  Gain=pass'  Multiplication=Matrix(K*u) (u vector)
  Gain8 : Gain  Gain=-1
  Gain9 : Gain  Gain=pass'  Multiplication=Matrix(K*u) (u vector)
  Integrator : Integrator
  Integrator1 : Integrator
  Mux : Mux  Inputs=[3 3]
  Mux1 : Mux  Inputs=[3 3]
  Mux2 : Mux  Inputs=[2 1]
  Mux3 : Mux  Inputs=[2 1]
  Mux4 : Mux  Inputs=3
  Mux5 : Mux  Inputs=[6 6 6]
  Sum : Sum  Inputs=|++
  Sum1 : Sum  Inputs=-+|
  Sum2 : Sum  Inputs=|++
  Sum4 : Sum  Inputs=++|
  "[0;0;0;ran]" : Gain  Gain=[zeros(3,1);ran]  Multiplication=Matrix(K*u) (u vector)
  "[0;0;0;ran]1" : Gain  Gain=[zeros(3,1);ran]  Multiplication=Matrix(K*u) (u vector)
  m_out|a : Outport  VectorParamsAs1DForOutWhenUnconnected=off
  W_r_in/.|p : Outport  Port=2  VectorParamsAs1DForOutWhenUnconnected=off
  m_theta : Outport  Port=3  VectorParamsAs1DForOutWhenUnconnected=off
  wires:
  18x18 v-u_rotation/1(y) -> m_out|a/1
  6x6 v-u_rotation/1(y) -> Demux/1
  Demux3/1 -> Mux2/1
  Demux2/1 -> Mux3/1
  Gain8/1 -> Mux3/2
  Mux3/1 -> Gain2/1
  Gain4/1 -> Demux3/1
  Demux1/2 -> Gain4/1
  Mux2/1 -> Gain3/1
  Demux2/2 -> Sum4/1
  Gain9/1 -> Demux2/1
  Demux3/2 -> Sum1/1
  Gain3/1 -> Mux/2
  Sum4/1 -> Gain1/1
  Gain1/1 -> Sum1/2, Mux2/2
  Demux/2 -> Gain9/1
  Gain2/1 -> Mux1/2
  Demux/1 -> Mux1/1
  Cm/1 -> Sum4/2, Gain8/1
  Demux1/1 -> Mux/1
  Mux1/1 -> W_r_in/.|p/1
  W_./r_out|a/1 -> 6x6 v-u_rotation/1(u)
  Demux4/1 -> Demux1/1
  m_in|p/1 -> Demux4/1
  Integrator/1 -> "[0;0;0;ran]"/1, Mux4/2, Integrator1/1
  Mux4/1 -> m_theta/1
  Sum1/1 -> Integrator/1, Mux4/1
  Integrator1/1 -> "[0;0;0;ran]1"/1, Mux4/3
  "[0;0;0;ran]"/1 -> Sum/2
  "[0;0;0;ran]1"/1 -> Sum2/2
  Demux4/2 -> Sum/1
  Demux4/3 -> Sum2/1
  Mux/1 -> Mux5/1
  Mux5/1 -> 18x18 v-u_rotation/1(u)
  Sum/1 -> Mux5/2
  Sum2/1 -> Mux5/3

== system FourFlexibleBarsFreeAug/TITOP bar #0 +revolute joint at P0=C3/Revolute joint + configuration/18x18 v-u_rotation ==
  u : Inport  PortDimensions=18
  Demux : Demux  Outputs=[3 3 3 3 3 3]
  Mux : Mux  Inputs=[3 3 3 3 3 3]
  Subsystem : Subsystem
  Subsystem1 : Subsystem
  Subsystem2 : Subsystem
  Subsystem3 : Subsystem
  Subsystem4 : Subsystem
  Subsystem5 : Subsystem
  y : Outport  VectorParamsAs1DForOutWhenUnconnected=off
  wires:
  Subsystem1/1(Out1) -> Mux/2
  Subsystem/1(Out1) -> Mux/1
  Demux/2 -> Subsystem1/1(In1)
  Demux/1 -> Subsystem/1(In1)
  u/1 -> Demux/1
  Mux/1 -> y/1
  Demux/3 -> Subsystem2/1(In1)
  Subsystem2/1(Out1) -> Mux/3
  Demux/4 -> Subsystem3/1(In1)
  Subsystem3/1(Out1) -> Mux/4
  Demux/5 -> Subsystem4/1(In1)
  Subsystem4/1(Out1) -> Mux/5
  Demux/6 -> Subsystem5/1(In1)
  Subsystem5/1(Out1) -> Mux/6

== system FourFlexibleBarsFreeAug/TITOP bar #0 +revolute joint at P0=C3/Revolute joint + configuration/6x6 v-u_rotation ==
  u : Inport  PortDimensions=6
  Demux : Demux  Outputs=[3 3]
  Mux : Mux  Inputs=[3 3]
  Subsystem : Subsystem
  Subsystem1 : Subsystem
  y : Outport  VectorParamsAs1DForOutWhenUnconnected=off
  wires:
  Mux/1 -> y/1
  u/1 -> Demux/1
  Demux/1 -> Subsystem/1(In1)
  Demux/2 -> Subsystem1/1(In1)
  Subsystem/1(Out1) -> Mux/1
  Subsystem1/1(Out1) -> Mux/2

== system FourFlexibleBarsFreeAug/TITOP bar #1 +revolute joint at C0=P1/Revolute joint + configuration/18x18 v-u_rotation ==
  u : Inport  PortDimensions=18
  Demux : Demux  Outputs=[3 3 3 3 3 3]
  Mux : Mux  Inputs=[3 3 3 3 3 3]
  Subsystem : Subsystem
  Subsystem1 : Subsystem
  Subsystem2 : Subsystem
  Subsystem3 : Subsystem
  Subsystem4 : Subsystem
  Subsystem5 : Subsystem
  y : Outport  VectorParamsAs1DForOutWhenUnconnected=off
  wires:
  Subsystem5/1(Out1) -> Mux/6
  Demux/6 -> Subsystem5/1(In1)
  Subsystem4/1(Out1) -> Mux/5
  Demux/5 -> Subsystem4/1(In1)
  Subsystem3/1(Out1) -> Mux/4
  Demux/4 -> Subsystem3/1(In1)
  Subsystem2/1(Out1) -> Mux/3
  Demux/3 -> Subsystem2/1(In1)
  Mux/1 -> y/1
  u/1 -> Demux/1
  Demux/1 -> Subsystem/1(In1)
  Demux/2 -> Subsystem1/1(In1)
  Subsystem/1(Out1) -> Mux/1
  Subsystem1/1(Out1) -> Mux/2

== system FourFlexibleBarsFreeAug/TITOP bar #1 +revolute joint at C0=P1/Revolute joint + configuration/6x6 v-u_rotation ==
  u : Inport  PortDimensions=6
  Demux : Demux  Outputs=[3 3]
  Mux : Mux  Inputs=[3 3]
  Subsystem : Subsystem
  Subsystem1 : Subsystem
  y : Outport  VectorParamsAs1DForOutWhenUnconnected=off
  wires:
  Subsystem1/1(Out1) -> Mux/2
  Subsystem/1(Out1) -> Mux/1
  Demux/2 -> Subsystem1/1(In1)
  Demux/1 -> Subsystem/1(In1)
  u/1 -> Demux/1
  Mux/1 -> y/1
